simulink subsystem "Field_Oriented_Control"  (R2022b)
settings: Solver=VariableStepAuto  StartTime=0.0  StopTime=10.0  RelTol=1e-3
model mask{AxisAlignment=D-axis}
  mask prompts: AxisAlignment "Alpha (phase-a) axis alignment:"
undefined symbols (not defined in the file): DiscIntNeverNeededParam, PI_params, pmsm, PU_System, T_cpu, Ts_speed
libraries: mcbcontrolslib x3
settings Model: Creator=The MathWorks, Inc.  LastModifiedBy=snarayan
settings SolverCC: AlgebraicLoopSolver=TrustRegion  MaxZcPerStep=1
settings DebuggingCC: UnconnectedInputMsg=warning  UnconnectedOutputMsg=warning  UnconnectedLineMsg=warning  SFMachineParentedDataDiag=warning
settings ModelReferenceCC: EnableRefExpFcnMdlSchedulingChecks=on
settings RTWCC: DLArmComputeVersion=19.05

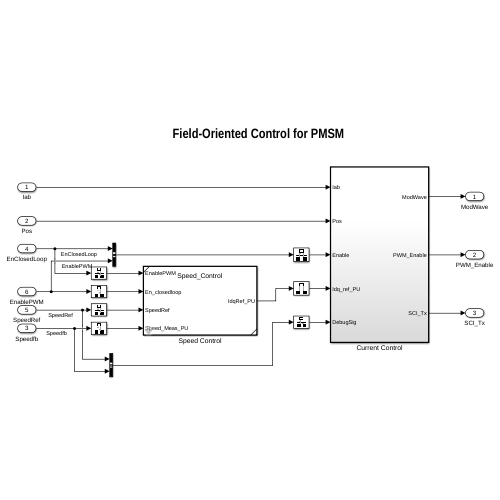
[thumbnail: Simulink's stored preview of the top-level diagram]
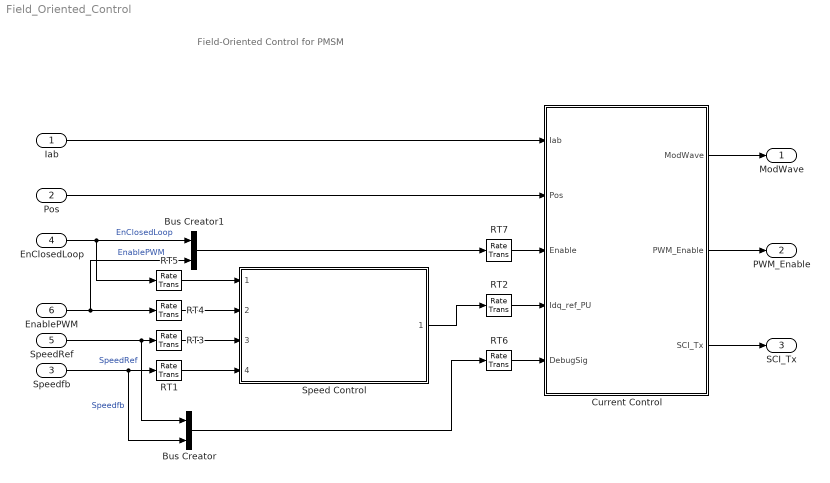
== system Field_Oriented_Control ==
  note: Field-Oriented Control for PMSM
  Iab : Inport
  Pos : Inport  Port=2
  Speedfb : Inport  Port=3
  EnClosedLoop : Inport  Port=4
  SpeedRef : Inport  Port=5
  EnablePWM : Inport  Port=6
  Bus Creator : BusCreator  Inputs=2
  Bus Creator1 : BusCreator  Inputs=2
  Current Control : Subsystem  TreatAsAtomicUnit=on
  RT{1,3..5} (4 alike) : RateTransition  Deterministic=off  OutPortSampleTime=Ts_speed
  RT2 : RateTransition  Deterministic=off
  RT6 : RateTransition  Deterministic=off
  RT7 : RateTransition  Deterministic=off
  Speed Control : Subsystem  TreatAsAtomicUnit=on  SystemSampleTime=Ts_speed  ReferencedSubsystem=Speed_Control  Kp_speed=PI_params.Kp_speed  Ki_speed=PI_params.Ki_speed*Ts_speed
  ModWave : Outport
  PWM_Enable : Outport  Port=2
  SCI_Tx : Outport  Port=3
  wires:
  Speedfb/1 -> RT1/1, Bus Creator/2  "Speedfb"
  RT1/1 -> Speed Control/4
  RT4/1 -> Speed Control/2
  SpeedRef/1 -> RT3/1, Bus Creator/1  "SpeedRef"
  EnablePWM/1 -> Bus Creator1/2, RT4/1  "EnablePWM"
  Speed Control/1 -> RT2/1
  RT3/1 -> Speed Control/3
  RT5/1 -> Speed Control/1
  Bus Creator/1 -> RT6/1
  EnClosedLoop/1 -> RT5/1, Bus Creator1/1  "EnClosedLoop"
  RT6/1 -> Current Control/5(DebugSig)
  RT2/1 -> Current Control/4(Idq_ref_PU)
  Pos/1 -> Current Control/2(Pos)
  Iab/1 -> Current Control/1(Iab)
  Bus Creator1/1 -> RT7/1
  Current Control/2(PWM_Enable) -> PWM_Enable/1
  Current Control/1(ModWave) -> ModWave/1
  Current Control/3(SCI_Tx) -> SCI_Tx/1
  RT7/1 -> Current Control/3(Enable)

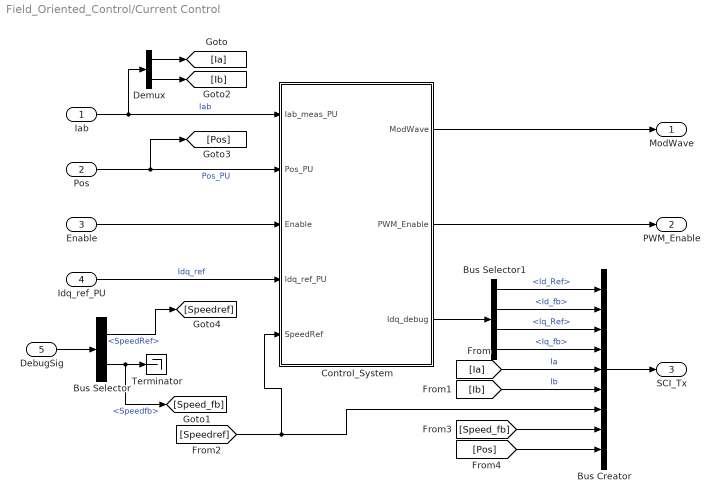
== system Field_Oriented_Control/Current Control ==
  Iab : Inport
  Pos : Inport  Port=2
  Enable : Inport  Port=3
  Idq_ref_PU : Inport  Port=4
  DebugSig : Inport  Port=5
  Bus Creator : BusCreator  Inputs=9
  Bus Selector : BusSelector  OutputSignals=SpeedRef,Speedfb
  Bus Selector1 : BusSelector  OutputSignals=Id_Ref,Id_fb,Iq_Ref,Iq_fb
  Control_System : Subsystem
  Demux : Demux  Outputs=2
  Terminator : Terminator
  ModWave : Outport  InitialOutput=0  VectorParamsAs1DForOutWhenUnconnected=off
  PWM_Enable : Outport  Port=2  InitialOutput=0  VectorParamsAs1DForOutWhenUnconnected=off
  SCI_Tx : Outport  Port=3
  wires:
  Demux/2 -> [Ib]
  Demux/1 -> [Ia]
  Bus Creator/1 -> SCI_Tx/1
  Control_System/2(PWM_Enable) -> PWM_Enable/1
  Control_System/1(ModWave) -> ModWave/1
  Bus Selector/2 -> [Speed_fb], Terminator/1  "<Speedfb>"
  Bus Selector/1 -> [Speedref]  "<SpeedRef>"
  DebugSig/1 -> Bus Selector/1
  Iab/1 -> Control_System/1(Iab_meas_PU), Demux/1  "Iab"
  Control_System/3(Idq_debug) -> Bus Selector1/1
  Enable/1 -> Control_System/3(Enable)
  Pos/1 -> [Pos], Control_System/2(Pos_PU)  "Pos_PU"
  Idq_ref_PU/1 -> Control_System/4(Idq_ref_PU)  "Idq_ref"
  Bus Selector1/1 -> Bus Creator/1  "<Id_Ref>"
  Bus Selector1/2 -> Bus Creator/2  "<Id_fb>"
  Bus Selector1/3 -> Bus Creator/3  "<Iq_Ref>"
  Bus Selector1/4 -> Bus Creator/4  "<Iq_fb>"
  [Ia] -> Bus Creator/5  "Ia"
  [Ib] -> Bus Creator/6  "Ib"
  [Speedref] -> Bus Creator/7, Control_System/5(SpeedRef)
  [Speed_fb] -> Bus Creator/8
  [Pos] -> Bus Creator/9

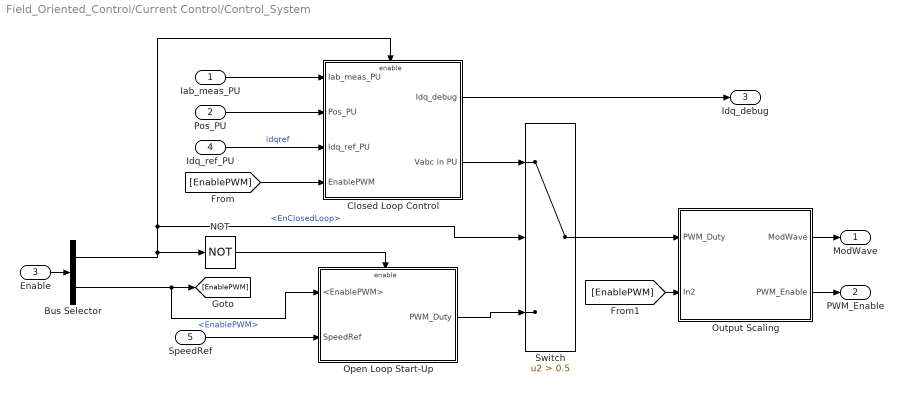
== system Field_Oriented_Control/Current Control/Control_System ==
  Iab_meas_PU : Inport
  Pos_PU : Inport  Port=2
  Enable : Inport  Port=3
  Idq_ref_PU : Inport  Port=4
  SpeedRef : Inport  Port=5
  Bus Selector : BusSelector  OutputSignals=EnClosedLoop,EnablePWM
  Closed Loop Control : Subsystem
  NOT : Logic  Operator=NOT  IconShape=distinctive  AllPortsSameDT=off  OutDataTypeStr=boolean
  Open Loop Start-Up : Subsystem
  Output Scaling : Subsystem
  Switch : Switch  Criteria=u2 > Threshold  Threshold=0.5  SaturateOnIntegerOverflow=off  InputSameDT=off
  ModWave : Outport
  PWM_Enable : Outport  Port=2
  Idq_debug : Outport  Port=3  VectorParamsAs1DForOutWhenUnconnected=off
  wires:
  SpeedRef/1 -> Open Loop Start-Up/2(SpeedRef)
  [EnablePWM] -> Output Scaling/2(In2)
  Output Scaling/2(PWM_Enable) -> PWM_Enable/1
  Output Scaling/1(ModWave) -> ModWave/1
  Closed Loop Control/2(Vabc in PU) -> Switch/1
  Closed Loop Control/1(Idq_debug) -> Idq_debug/1
  [EnablePWM] -> Closed Loop Control/4(EnablePWM)
  Idq_ref_PU/1 -> Closed Loop Control/3(Idq_ref_PU)  "idqref"
  Pos_PU/1 -> Closed Loop Control/2(Pos_PU)
  Iab_meas_PU/1 -> Closed Loop Control/1(Iab_meas_PU)
  Bus Selector/2 -> [EnablePWM], Open Loop Start-Up/1(<EnablePWM>)  "<EnablePWM>"
  Bus Selector/1 -> NOT/1, Switch/2, Closed Loop Control/Enable  "<EnClosedLoop>"
  Enable/1 -> Bus Selector/1
  NOT/1 -> Open Loop Start-Up/Enable
  Switch/1 -> Output Scaling/1(PWM_Duty)
  Open Loop Start-Up/1(PWM_Duty) -> Switch/3

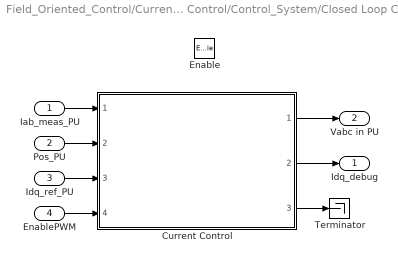
== system Field_Oriented_Control/Current Control/Control_System/Closed Loop Control ==
  Iab_meas_PU : Inport
  Pos_PU : Inport  Port=2
  Idq_ref_PU : Inport  Port=3
  EnablePWM : Inport  Port=4
  Enable : EnablePort
  Current Control : Subsystem  ReferencedSubsystem=Current_Control  Kpd=PI_params.Kp_i  Kid=PI_params.Ki_i*T_cpu  Kpq=PI_params.Kp_i  Kiq=PI_params.Ki_i*T_cpu
  Terminator : Terminator
  Idq_debug : Outport
  Vabc in PU : Outport  Port=2
  wires:
  Current Control/1 -> Vabc in PU/1
  Current Control/2 -> Idq_debug/1
  Pos_PU/1 -> Current Control/2
  EnablePWM/1 -> Current Control/4
  Iab_meas_PU/1 -> Current Control/1
  Idq_ref_PU/1 -> Current Control/3
  Current Control/3 -> Terminator/1

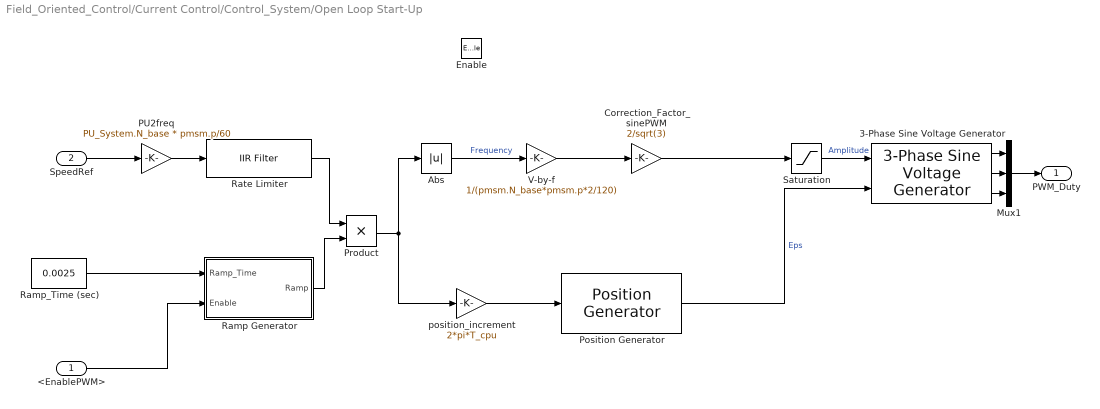
== system Field_Oriented_Control/Current Control/Control_System/Open Loop Start-Up ==
  <EnablePWM> : Inport
  SpeedRef : Inport  Port=2
  Enable : EnablePort
  3-Phase Sine Voltage Generator : mcbcontrolslib/3-Phase Sine Voltage Generator  AngleInput=Radians  N_points=1024
  Abs : Abs  SaturateOnIntegerOverflow=off
  Correction_Factor_sinePWM : Gain  Gain=2/sqrt(3)  RndMeth=Simplest  OutDataTypeStr=Inherit: Same as input
  Mux1 : Mux  Inputs=3
  PU2freq : Gain  Gain=PU_System.N_base * pmsm.p/60  RndMeth=Simplest  OutDataTypeStr=Inherit: Same as input
  Position Generator : mcbcontrolslib/Position Generator  AngleOutput=Radians  ThetaSource=External  ThetaInput=5e-4  DataType=double  ExternalReset=none  Offset=0
  Product : Product  RndMeth=Simplest  OutDataTypeStr=Inherit: Same as first input
  Ramp Generator : Subsystem
  Ramp_Time (sec) : Constant  Value=0.0025  OutDataTypeStr=dataType  SampleTime=-1
  Rate Limiter : mcbcontrolslib/IIR Filter  VariantControl=Low Pass Filter  VariantSelect=Low-pass  Filter_constant=0.0001  advancedSettings=off  Ts=50e-6  cutOff_freq=0.31834
  Saturation : Saturate  UpperLimit=0.95  LowerLimit=0.15  RndMeth=Simplest
  V-by-f : Gain  Gain=1/(pmsm.N_base*pmsm.p*2/120)  RndMeth=Simplest  OutDataTypeStr=Inherit: Same as input
  position_increment : Gain  Gain=2*pi*T_cpu  RndMeth=Simplest  OutDataTypeStr=Inherit: Same as input
  PWM_Duty : Outport  VectorParamsAs1DForOutWhenUnconnected=off
  wires:
  SpeedRef/1 -> PU2freq/1
  Rate Limiter/1 -> Product/1
  Product/1 -> position_increment/1, Abs/1
  <EnablePWM>/1 -> Ramp Generator/2(Enable)
  3-Phase Sine Voltage Generator/2 -> Mux1/2
  Correction_Factor_sinePWM/1 -> Saturation/1
  PU2freq/1 -> Rate Limiter/1
  V-by-f/1 -> Correction_Factor_sinePWM/1
  position_increment/1 -> Position Generator/1
  Abs/1 -> V-by-f/1  "Frequency"
  Ramp_Time (sec)/1 -> Ramp Generator/1(Ramp_Time)
  Ramp Generator/1(Ramp) -> Product/2
  Mux1/1 -> PWM_Duty/1
  Saturation/1 -> 3-Phase Sine Voltage Generator/1  "Amplitude"
  Position Generator/1 -> 3-Phase Sine Voltage Generator/2  "Eps"
  3-Phase Sine Voltage Generator/3 -> Mux1/3
  3-Phase Sine Voltage Generator/1 -> Mux1/1

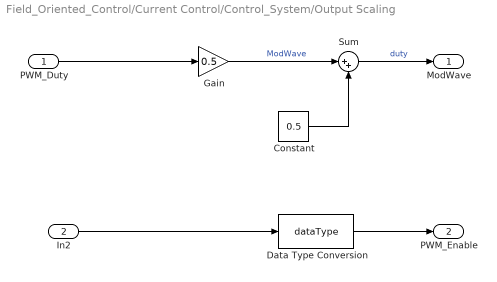
== system Field_Oriented_Control/Current Control/Control_System/Output Scaling ==
  PWM_Duty : Inport
  In2 : Inport  Port=2
  Constant : Constant  Value=0.5  OutDataTypeStr=dataType
  Data Type Conversion : DataTypeConversion  OutDataTypeStr=dataType  SaturateOnIntegerOverflow=off  RndMeth=Floor
  Gain : Gain  Gain=0.5  OutDataTypeStr=Inherit: Same as input
  Sum : Sum  Inputs=|++
  ModWave : Outport
  PWM_Enable : Outport  Port=2
  wires:
  In2/1 -> Data Type Conversion/1
  Data Type Conversion/1 -> PWM_Enable/1
  PWM_Duty/1 -> Gain/1
  Gain/1 -> Sum/1  "ModWave"
  Constant/1 -> Sum/2
  Sum/1 -> ModWave/1  "duty"

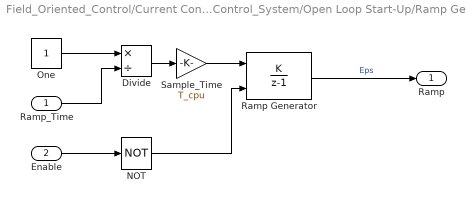
== system Field_Oriented_Control/Current Control/Control_System/Open Loop Start-Up/Ramp Generator ==
  Ramp_Time : Inport
  Enable : Inport  Port=2
  Divide : Product  Inputs=*/  RndMeth=Simplest  OutDataTypeStr=Inherit: Same as first input
  NOT : Logic  Operator=NOT  IconShape=distinctive  AllPortsSameDT=off  OutDataTypeStr=boolean
  One : Constant  OutDataTypeStr=dataType  SampleTime=-1
  Ramp Generator : DiscreteIntegrator  IntegratorMethod=Accumulation: Forward Euler  gainval=1  ExternalReset=sampled level  SampleTime=-1  OutDataTypeStr=dataType  RndMeth=Simplest  LimitOutput=on  UpperSaturationLimit=1  LowerSaturationLimit=0  ICPrevOutput=DiscIntNeverNeededParam  ICPrevScaledInput=DiscIntNeverNeededParam
  Sample_Time : Gain  Gain=T_cpu  RndMeth=Simplest  OutDataTypeStr=Inherit: Same as input
  Ramp : Outport
  wires:
  NOT/1 -> Ramp Generator/2
  Enable/1 -> NOT/1
  Ramp_Time/1 -> Divide/2
  One/1 -> Divide/1
  Sample_Time/1 -> Ramp Generator/1
  Ramp Generator/1 -> Ramp/1  "Eps"
  Divide/1 -> Sample_Time/1
